simulink model "convert_Voltage_to_Current"  (R2021a)
settings: Solver=VariableStepAuto  StartTime=0.0  StopTime=10.0  RelTol=1e-3
settings Model: Creator=HP  LastModifiedBy=HP

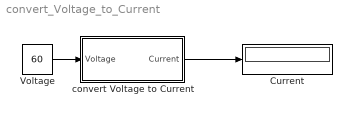
== system convert_Voltage_to_Current ==
  " convert Voltage to Current" : Subsystem
  Current : Display
  Voltage : Constant  Value=60
  wires:
  " convert Voltage to Current"/1(Current) -> Current/1
  Voltage/1 -> " convert Voltage to Current"/1(Voltage)

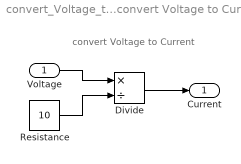
== system convert_Voltage_to_Current/ convert Voltage to Current ==
  note: convert Voltage to Current
  Voltage : Inport
  Divide : Product  Inputs=*/
  Resistance : Constant  Value=10
  Current : Outport
  wires:
  Voltage/1 -> Divide/1
  Resistance/1 -> Divide/2
  Divide/1 -> Current/1
